simulink library "sumAttchPtsFnM_ul"  (R2018b)
settings: Solver=VariableStepAuto  StartTime=0.0  StopTime=10.0  RelTol=1e-3
undefined symbols (not defined in the file or in its folder): class_thr
libraries: vrlib x1, eulAng2RotMat_ul x1
settings Model: Creator=Ayaz  LastModifiedBy=asiddiq2

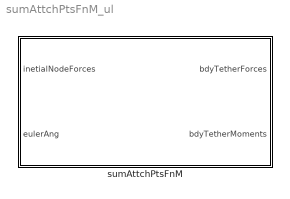
== system sumAttchPtsFnM_ul ==
  sumAttchPtsFnM : Subsystem  TreatAsAtomicUnit=on  mask{cls_obj=class_thr}
      mask prompts: cls_obj "Object consisting attachment points"

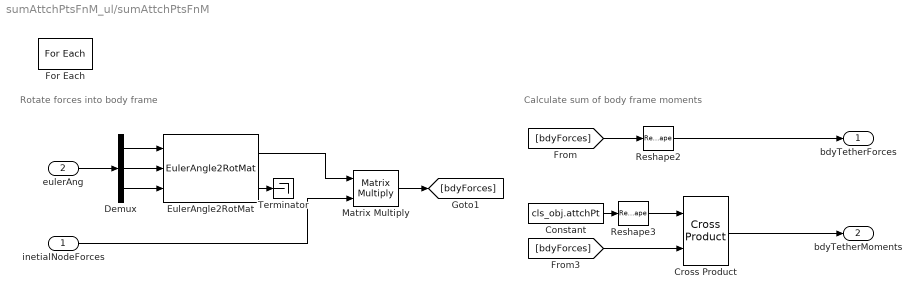
== system sumAttchPtsFnM_ul/sumAttchPtsFnM ==
  note: Rotate forces into body frame
  note: Calculate sum of body frame moments
  inetialNodeForces : Inport  Partition=on  PartitionDimension=2  PartitionWidth=1  PartitionOffset=0
  eulerAng : Inport  Port=2
  Constant : Constant  Value=cls_obj.attchPt  VectorParams1D=off
  Cross Product : vrlib/Utilities/Cross Product
      settings: SourceProductBaseCode=VR
  Demux : Demux  Outputs=3
  EulerAngle2RotMat : eulAng2RotMat_ul/EulerAngle2RotMat  SystemSampleTime=-1
  For Each : ForEach  DisableCoverage=on  IterateSubsysMaskParameter=on  SubsysMaskParameterIterationDimension=2  IndexMode=One-based
  Matrix Multiply : Product  Multiplication=Matrix(*)
  Reshape2 : Reshape  OutputDimensionality=Column vector (2-D)
  Reshape3 : Reshape  OutputDimensionality=Column vector (2-D)
  Terminator : Terminator
  bdyTetherForces : Outport  ConcatenationDimension=2
  bdyTetherMoments : Outport  Port=2  ConcatenationDimension=2
  wires:
  EulerAngle2RotMat/1 -> Matrix Multiply/1
  Demux/1 -> EulerAngle2RotMat/1
  EulerAngle2RotMat/2 -> Terminator/1
  inetialNodeForces/1 -> Matrix Multiply/2
  Demux/2 -> EulerAngle2RotMat/2
  Demux/3 -> EulerAngle2RotMat/3
  Matrix Multiply/1 -> [bdyForces]
  eulerAng/1 -> Demux/1
  Cross Product/1 -> bdyTetherMoments/1
  [bdyForces] -> Cross Product/2
  Constant/1 -> Reshape3/1
  [bdyForces] -> Reshape2/1
  Reshape2/1 -> bdyTetherForces/1
  Reshape3/1 -> Cross Product/1
